simulink model "ddc_bpm_hw_cosim"  (Simulink 7.8)
settings: Solver=ode45  StartTime=0.0  StopTime=6e-4  RelTol=1e-3
undefined symbols (not defined in the file): A, Fs_adc, Fs_adc_image, N
libraries: simulink x2, xbsIndex_r4 x1, JTAGRuntimeCosim_r4 x1
settings Model: Creator=lucas.russo  LastModifiedBy=lucas.russo

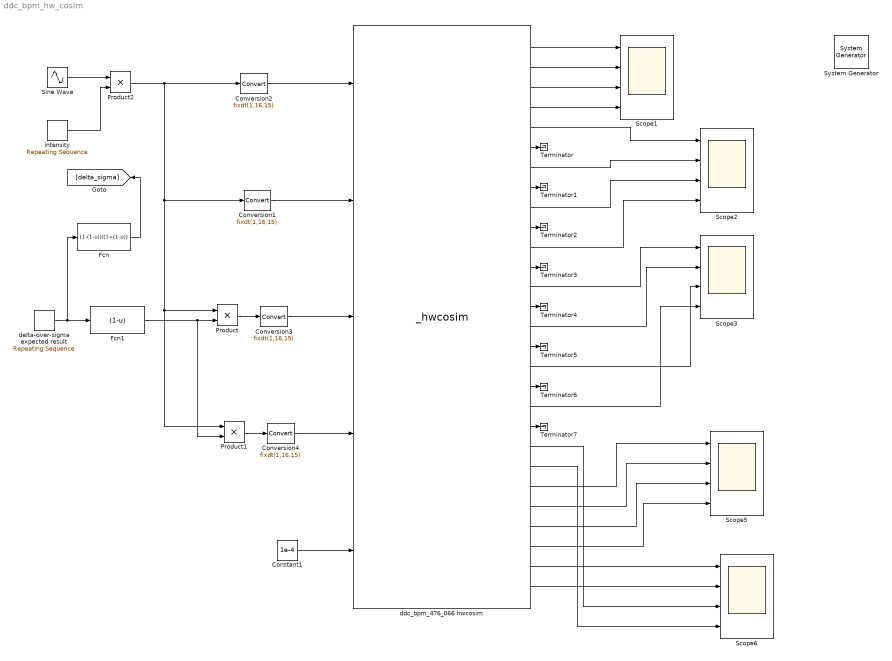
== system ddc_bpm_hw_cosim ==
  " System Generator" : xbsIndex_r4/ System Generator  Tag=genX  xilinxfamily=virtex6  part=xc6vlx240t  speed=-1  package=ff1156  synthesis_tool=XST  clock_wrapper=Clock Enables  directory=./netlistJTAG_COsim_ddc_bpm_476_066  proj_type=Project Navigator  Synth_file=XST Defaults  Impl_file=ISE Defaults  testbench=on  simulink_period=dt_sim  sysclk_period=10  dcm_input_clock_period=10  incr_netlist=off  trim_vbits=Everywhere in SubSystem  dbl_ovrd=According to Block Masks  core_generation=According to Block Masks  run_coregen=off  deprecated_control=off  eval_field=0  block_type=sysgen
  Constant1 : Constant  Value=1e-4  OutDataTypeStr=fixdt(1,26,22)
  Conversion{1..4} (4 alike) : DataTypeConversion  OutDataTypeStr=fixdt(1,16,15)  ConvertRealWorld=Stored Integer (SI)  LockScale=on
  Fcn : Fcn  Expr=(1-(1-u))/(1+(1-u))
  Fcn1 : Fcn  Expr=(1-u)
  Product : Product  RndMeth=Zero
  Product1 : Product  RndMeth=Zero
  Product2 : Product  RndMeth=Zero
  Scope{1..3,5..6} (5 alike) : Scope  NumInputPorts=4
      Scope1 settings: TimeRange=4.726537192257835e-007  YMin=4.34876e-005~0.463882~0.00990226~4.5e-005  YMax=4.80652e-005~0.512712~0.0111025~9.5e-005  MaxDataPoints=1000000
      Scope2 settings: TimeRange=4.726537192257835e-007  YMin=4.34876e-005~0.463882~0.00990226~4.5e-005  YMax=4.80652e-005~0.512712~0.0111025~9.5e-005  MaxDataPoints=1000000
      Scope3 settings: TimeRange=4.726537192257835e-007  YMin=4.34876e-005~0.463882~0.00990226~4.5e-005  YMax=4.80652e-005~0.512712~0.0111025~9.5e-005  SaveName=ScopeData2  MaxDataPoints=1000000
      Scope5 settings: TimeRange=4.726537192257835e-007  YMin=4.34876e-005~0.463882~0.00990226~4.5e-005  YMax=4.80652e-005~0.512712~0.0111025~9.5e-005  SaveName=ScopeData4  MaxDataPoints=1000000
      Scope6 settings: TimeRange=4.726537192257835e-007  YMin=4.34876e-005~0.463882~0.00990226~4.5e-005  YMax=4.80652e-005~0.512712~0.0111025~9.5e-005  SaveName=ScopeData5  MaxDataPoints=1000000
  Sine Wave : Sin  Amplitude=2^(16-1)  Frequency=2*pi*Fs_adc_image  SampleTime=1/Fs_adc
  Terminator{,1..7} (8 alike) : Terminator
  ddc_bpm_476_066 hwcosim : JTAGRuntimeCosim_r4/_hwcosim  clkSrc=Single Stepped  hasCombinationalPath=on  bitfileName=D:\Sysgen_projects\ddc_bpm_476_066\models\netlistJTAG_COsim_ddc_bpm_476_066\ddc_bpm_476_066_cw.bit  skipConfig=off  cable=Auto Detect  speed=N/A  cablePort=N/A  cableLocation=Local  shareCable=off  enable_codebug=on  design_xtable=|  engineDll=JTAGCosimEngine.dll  cableWaitTime=10  bscanPos=-1  IRLengths=[]  useWaitBox=1  hasBufgmux=on  Scheme=Cosim  useCmdProc=1  hasProc=0  block_type=jtagcosim
      | {
      |   'clkWrapper' => 'ddc_bpm_476_066_cw',
      |   'clocksGcd' => 1,
      |   'device' => 'xc6vlx240t-1ff1156',
      |   'ports' => {
      |     'adc_ch0_i' => {
      |       'bd_port_index' => 0,
      |       'direction' => 'in',
      |       'icon_text' => 'adc_ch0_i',
      |       'period' => 1,
      |       'proxy_name' => 'ddc_bpm_476_066/Channel0/adc_ch0_i',
      |       'sim_pause_trigger' => false,
      |       'type' => 'Fix_16_15',
      |       'width' => 16,
      |     },
      |     'adc_ch1_i' => {
      |       'bd_port_index' => 1,
      |       'direction' => 'in',
      |       'icon_text' => 'adc_ch1_i',
      |       'period' => 1,
      |       'proxy_name' => 'ddc_bpm_476_066/Channel1/adc_ch1_i',
      |       'sim_pause_trigger' => false,
      |       'type' => 'Fix_16_15',
      |       'width' => 16,
      |     },
      |     'adc_ch2_i' => {
      |       'bd_port_index' => 2,
      |       'direction' => 'in',
      |       'icon_text' => 'adc_ch2_i',
      |       'period' => 1,
      |       'proxy_name' => 'ddc_bpm_476_066/Channel2/adc_ch2_i',
      |       'sim_pause_trigger' => false,
      |       'type' => 'Fix_16_15',
      |       'width' => 16,
      |     },
      |     'adc_ch3_i' => {
      |       'bd_port_index' => 3,
      |       'direction' => 'in',
      |       'icon_text' => 'adc_ch3_i',
      |       'period' => 1,
      |       'proxy_name' => 'ddc_bpm_476_066/Channel3/adc_ch3_i',
      |       'sim_pause_trigger' => false,
      |       'type' => 'Fix_16_15',
      |       'width' => 16,
      |     },
      |     'bpf_ch0_o' => {
      |       'bd_port_index' => 0,
      |       'direction' => 'out',
      |       'icon_text' => 'bpf_ch0_o',
      |       'period' => 1,
      |       'proxy_name' => 'ddc_bpm_476_066/Channel0/bpf_ch0_o',
      |       'sim_pause_trigger' => false,
      |       'type' => 'Fix_24_22',
      |       'width' => 24,
      |     },
      |     'bpf_ch1_o' => {
      |       'bd_port_index' => 1,
      |       'direction' => 'out',
      |       'icon_text' => 'bpf_ch1_o',
      |       'period' => 1,
      |       'proxy_name' => 'ddc_bpm_476_066/Channel1/bpf_ch1_o',
      |       'sim_pause_trigger' => false,
      |       'type' => 'Fix_24_22',
      |       'width' => 24,
      |     },
      |     'bpf_ch2_o' => {
      |       'bd_port_index' => 2,
      |       'direction' => 'out',
      |       'icon_text' => 'bpf_ch2_o',
      |       'period' => 1,
      |       'proxy_name' => 'ddc_bpm_476_066/Channel2/bpf_ch2_o',
      |       'sim_pause_trigger' => false,
      |       'type' => 'Fix_24_22',
      |       'width' => 24,
      |     },
      |     'bpf_ch3_o' => {
      |       'bd_port_index' => 3,
      |       'direction' => 'out',
      |       'icon_text' => 'bpf_ch3_o',
      |       'period' => 1,
      |       'proxy_name' => 'ddc_bpm_476_066/Channel3/bpf_ch3_o',
      |       'sim_pause_trigger' => false,
      |       'type' => 'Fix_24_22',
      |       'width' => 24,
      |     },
      |     'del_sig_div_thres_i' => {
      |       'bd_port_index' => 4,
      |       'direction' => 'in',
      |       'icon_text' => 'del_sig_div_thres_i',
      |       'period' => 1,
      |       'proxy_name' => 'ddc_bpm_476_066/del_sig_div_thres_i',
      |       'sim_pause_trigger' => false,
      |       'type' => 'Fix_16_15',
      |       'width' => 16,
      |     },
      |     'mix_ch0_i_o' => {
      |       'bd_port_index' => 4,
      |       'direction' => 'out',
      |       'icon_text' => 'mix_ch0_i_o',
      |       'period' => 1,
      |       'proxy_name' => 'ddc_bpm_476_066/Channel0/mix_ch0_i_o',
      |       'sim_pause_trigger' => false,
      |       'type' => 'Fix_24_22',
      |       'width' => 24,
      |     },
      |     'mix_ch0_q_o' => {
      |       'bd_port_index' => 5,
      |       'direction' => 'out',
      |       'icon_text' => 'mix_ch0_q_o',
      |       'period' => 1,
      |       'proxy_name' => 'ddc_bpm_476_066/Channel0/mix_ch0_q_o',
      |       'sim_pause_trigger' => false,
      |       'type' => 'Fix_24_22',
      |       'width' => 24,
      |     },
      |     'mix_ch1_i_o' => {
      |       'bd_port_index' => 6,
      |       'direction' => 'out',
      |       'icon_text' => 'mix_ch1_i_o',
      |       'period' => 1,
      |       'proxy_name' => 'ddc_bpm_476_066/Channel1/mix_ch1_i_o',
      |       'sim_pause_trigger' => false,
      |       'type' => 'Fix_24_22',
      |       'width' => 24,
      |     },
      |     'mix_ch1_q_o' => {
      |       'bd_port_index' => 7,
      |       'direction' => 'out',
      |       'icon_text' => 'mix_ch1_q_o',
      |       'period' => 1,
      |       'proxy_name' => 'ddc_bpm_476_066/Channel1/mix_ch1_q_o',
      |       'sim_pause_trigger' => false,
      |       'type' => 'Fix_24_22',
      |       'width' => 24,
      |     },
      |     'mix_ch2_i_o' => {
      |       'bd_port_index' => 8,
      |       'direction' => 'out',
      |       'icon_text' => 'mix_ch2_i_o',
      |       'period' => 1,
      |       'proxy_name' => 'ddc_bpm_476_066/Channel2/mix_ch2_i_o',
      |       'sim_pause_trigger' => false,
      |       'type' => 'Fix_24_22',
      |       'width' => 24,
      |     },
      |     'mix_ch2_q_o' => {
      |       'bd_port_index' => 9,
      |       'direction' => 'out',
      |       'icon_text' => 'mix_ch2_q_o',
      |       'period' => 1,
      |       'proxy_name' => 'ddc_bpm_476_066/Channel2/mix_ch2_q_o',
      |       'sim_pause_trigger' => false,
      |       'type' => 'Fix_24_22',
      |       'width' => 24,
      |     },
      |     'mix_ch3_i_o' => {
      |       'bd_port_index' => 10,
      |       'direction' => 'out',
      |       'icon_text' => 'mix_ch3_i_o',
      |       'period' => 1,
      |       'proxy_name' => 'ddc_bpm_476_066/Channel3/mix_ch3_i_o',
      |       'sim_pause_trigger' => false,
      |       'type' => 'Fix_24_22',
      |       'width' => 24,
      |     },
      |     'mix_ch3_q_o' => {
      |       'bd_port_index' => 11,
      |       'direction' => 'out',
      |       'icon_text' => 'mix_ch3_q_o',
      |       'period' => 1,
      |       'proxy_name' => 'ddc_bpm_476_066/Channel3/mix_ch3_q_o',
      |       'sim_pause_trigger' => false,
      |       'type' => 'Fix_24_22',
      |       'width' => 24,
      |     },
      |     'poly35_ch0_i_o' => {
      |       'bd_port_index' => 12,
      |       'direction' => 'out',
      |       'icon_text' => 'poly35_ch0_i_o',
      |       'period' => 35,
      |       'proxy_name' => 'ddc_bpm_476_066/Channel0/poly35_ch0_i_o',
      |       'sim_pause_trigger' => false,
      |       'type' => 'Fix_24_22',
      |       'width' => 24,
      |     },
      |     'poly35_ch0_q_o' => {
      |       'bd_port_index' => 13,
      |       'direction' => 'out',
      |       'icon_text' => 'poly35_ch0_q_o',
      |       'period' => 35,
      |       'proxy_name' => 'ddc_bpm_476_066/Channel0/poly35_ch0_q_o',
      |       'sim_pause_trigger' => false,
      |       'type' => 'Fix_24_22',
      |       'width' => 24,
      |     },
      |     'poly35_ch1_i_o' => {
      |       'bd_port_index' => 14,
      |       'direction' => 'out',
      |       'icon_text' => 'poly35_ch1_i_o',
      |       'period' => 35,
      |       'proxy_name' => 'ddc_bpm_476_066/Channel1/poly35_ch1_i_o',
      |       'sim_pause_trigger' => false,
      |       'type' => 'Fix_24_22',
      |       'width' => 24,
      |     },
      |     'poly35_ch1_q_o' => {
      |       'bd_port_index' => 15,
      |       'direction' => 'out',
      |       'icon_text' => 'poly35_ch1_q_o',
      |       'period' => 35,
      |       'proxy_name' => 'ddc_bpm_476_066/Channel1/poly35_ch1_q_o',
      |       'sim_pause_trigger' => false,
      |       'type' => 'Fix_24_22',
      |       'width' => 24,
      |     },
      |     'poly35_ch2_i_o' => {
      |       'bd_port_index' => 16,
      |       'direction' => 'out',
      |       'icon_text' => 'poly35_ch2_i_o',
      |       'period' => 35,
      |       'proxy_name' => 'ddc_bpm_476_066/Channel2/poly35_ch2_i_o',
      |       'sim_pause_trigger' => false,
      |       'type' => 'Fix_24_22',
      |       'width' => 24,
      |     },
      |     'poly35_ch2_q_o' => {
      |       'bd_port_index' => 17,
      |       'direction' => 'out',
      |       'icon_text' => 'poly35_ch2_q_o',
      |       'period' => 35,
      |       'proxy_name' => 'ddc_bpm_476_066/Channel2/poly35_ch2_q_o',
      |       'sim_pause_trigger' => false,
      |       'type' => 'Fix_24_22',
      |       'width' => 24,
      |     },
      |     'poly35_ch3_i_o' => {
      |       'bd_port_index' => 18,
      |       'direction' => 'out',
      |       'icon_text' => 'poly35_ch3_i_o',
      |       'period' => 35,
      |       'proxy_name' => 'ddc_bpm_476_066/Channel3/poly35_ch3_i_o',
      |       'sim_pause_trigger' => false,
      |       'type' => 'Fix_24_22',
      |       'width' => 24,
      |     },
      |     'poly35_ch3_q_o' => {
      |       'bd_port_index' => 19,
      |       'direction' => 'out',
      |       'icon_text' => 'poly35_ch3_q_o',
      |       'period' => 35,
      |       'proxy_name' => 'ddc_bpm_476_066/Channel3/poly35_ch3_q_o',
      |       'sim_pause_trigger' => false,
      |       'type' => 'Fix_24_22',
      |       'width' => 24,
      |     },
      |     'q_tbt_o' => {
      |       'bd_port_index' => 20,
      |       'direction' => 'out',
      |       'icon_text' => 'q_tbt_o',
      |       'period' => 1,
      |       'proxy_name' => 'ddc_bpm_476_066/q_tbt_o',
      |       'sim_pause_trigger' => false,
      |       'type' => 'Fix_22_22',
      |       'width' => 22,
      |     },
      |     'sum_tbt_o' => {
      |       'bd_port_index' => 21,
      |       'direction' => 'out',
      |       'icon_text' => 'sum_tbt_o',
      |       'period' => 1,
      |       'proxy_name' => 'ddc_bpm_476_066/sum_tbt_o',
      |       'sim_pause_trigger' => false,
      |       'type' => 'Fix_26_22',
      |       'width' => 26,
      |     },
      |     'tbt_amp_ch0_o' => {
      |       'bd_port_index' => 22,
      |       'direction' => 'out',
      |       'icon_text' => 'tbt_amp_ch0_o',
      |       'period' => 35,
      |       'proxy_name' => 'ddc_bpm_476_066/Channel0/tbt_amp_ch0_o',
      |       'sim_pause_trigger' => false,
      |       'type' => 'Fix_24_22',
      |       'width' => 24,
      |     },
      |     'tbt_amp_ch1_o' => {
      |       'bd_port_index' => 23,
      |       'direction' => 'out',
      |       'icon_text' => 'tbt_amp_ch1_o',
      |       'period' => 35,
      |       'proxy_name' => 'ddc_bpm_476_066/Channel1/tbt_amp_ch1_o',
      |       'sim_pause_trigger' => false,
      |       'type' => 'Fix_24_22',
      |       'width' => 24,
      |     },
      |     'tbt_amp_ch2_o' => {
      |       'bd_port_index' => 24,
      |       'direction' => 'out',
      |       'icon_text' => 'tbt_amp_ch2_o',
      |       'period' => 35,
      |       'proxy_name' => 'ddc_bpm_476_066/Channel2/tbt_amp_ch2_o',
      |       'sim_pause_trigger' => false,
      |       'type' => 'Fix_24_22',
      |       'width' => 24,
      |     },
      |     'tbt_amp_ch3_o' => {
      |       'bd_port_index' => 25,
      |       'direction' => 'out',
      |       'icon_text' => 'tbt_amp_ch3_o',
      |       'period' => 35,
      |       'proxy_name' => 'ddc_bpm_476_066/Channel3/tbt_amp_ch3_o',
      |       'sim_pause_trigger' => false,
      |       'type' => 'Fix_24_22',
      |       'width' => 24,
      |     },
      |     'x_tbt_o' => {
      |       'bd_port_index' => 26,
      |       'direction' => 'out',
      |       'icon_text' => 'x_tbt_o',
      |       'period' => 1,
      |       'proxy_name' => 'ddc_bpm_476_066/x_tbt_o',
      |       'sim_pause_trigger' => false,
      |       'type' => 'Fix_22_22',
      |       'width' => 22,
      |     },
      |     'y_tbt_o' => {
      |       'bd_port_index' => 27,
      |       'direction' => 'out',
      |       'icon_text' => 'y_tbt_o',
      |       'period' => 1,
      |       'proxy_name' => 'ddc_bpm_476_066/y_tbt_o',
      |       'sim_pause_trigger' => false,
      |       'type' => 'Fix_22_22',
      |       'width' => 22,
      |     },
      |   },
      |   'shared_memories' => {},
      | }
  delta-over-sigma expected result : simulink/Sources/Repeating Sequence  rep_seq_t=[0 0.25e-4 0.25e-4 0.5e-4 0.5e-4 0.75e-4 0.75e-4 1e-4]  rep_seq_y=[1e-4 1e-4 2e-4 2e-4 4e-4 4e-4 8e-4 8e-4]
  intensity : simulink/Sources/Repeating Sequence  rep_seq_t=[0 1e-4 1e-4 2e-4 2e-4 3e-4 3e-4 4e-4]  rep_seq_y=[1 1 0.1 0.1 0.01 0.01 0.001 0.001]
  wires:
  ddc_bpm_476_066 hwcosim/1 -> Scope1/1
  ddc_bpm_476_066 hwcosim/2 -> Scope1/2
  ddc_bpm_476_066 hwcosim/3 -> Scope1/3
  ddc_bpm_476_066 hwcosim/4 -> Scope1/4
  ddc_bpm_476_066 hwcosim/5 -> Scope2/1
  ddc_bpm_476_066 hwcosim/7 -> Scope2/2
  ddc_bpm_476_066 hwcosim/9 -> Scope2/3
  ddc_bpm_476_066 hwcosim/11 -> Scope2/4
  ddc_bpm_476_066 hwcosim/13 -> Scope3/1
  ddc_bpm_476_066 hwcosim/15 -> Scope3/2
  ddc_bpm_476_066 hwcosim/17 -> Scope3/3
  ddc_bpm_476_066 hwcosim/19 -> Scope3/4
  ddc_bpm_476_066 hwcosim/23 -> Scope5/1
  ddc_bpm_476_066 hwcosim/24 -> Scope5/2
  ddc_bpm_476_066 hwcosim/25 -> Scope5/3
  ddc_bpm_476_066 hwcosim/26 -> Scope5/4
  ddc_bpm_476_066 hwcosim/27 -> Scope6/1
  ddc_bpm_476_066 hwcosim/28 -> Scope6/2
  ddc_bpm_476_066 hwcosim/21 -> Scope6/3
  ddc_bpm_476_066 hwcosim/22 -> Scope6/4
  Product/1 -> Conversion3/1
  Sine Wave/1 -> Product2/1
  Product2/1 -> Conversion2/1, Conversion1/1, Product/1, Product1/1
  intensity/1 -> Product2/2
  delta-over-sigma expected result/1 -> Fcn/1, Fcn1/1
  Fcn/1 -> [delta_sigma]
  Conversion2/1 -> ddc_bpm_476_066 hwcosim/1
  Conversion1/1 -> ddc_bpm_476_066 hwcosim/2
  Fcn1/1 -> Product/2, Product1/2
  Conversion3/1 -> ddc_bpm_476_066 hwcosim/3
  Conversion4/1 -> ddc_bpm_476_066 hwcosim/4
  Product1/1 -> Conversion4/1
  Constant1/1 -> ddc_bpm_476_066 hwcosim/5
  ddc_bpm_476_066 hwcosim/6 -> Terminator/1
  ddc_bpm_476_066 hwcosim/8 -> Terminator1/1
  ddc_bpm_476_066 hwcosim/10 -> Terminator2/1
  ddc_bpm_476_066 hwcosim/12 -> Terminator3/1
  ddc_bpm_476_066 hwcosim/14 -> Terminator4/1
  ddc_bpm_476_066 hwcosim/16 -> Terminator5/1
  ddc_bpm_476_066 hwcosim/18 -> Terminator6/1
  ddc_bpm_476_066 hwcosim/20 -> Terminator7/1
